simulink model "pllEncoder"  (R2024b)
settings: Solver=FixedStepAuto  StartTime=0.0  StopTime=Tend  FixedStep=0.0001  RelTol=1e-4
values from neighbouring files (symbols this model uses):
  pole_1_Hz = -10    [computing_speed.m]    (also in setup.m)
  pole_2_Hz = -100    [computing_speed.m]    (also in setup.m)
  Ts = 1e-4    (= 0.0001)    [setup.m]    (also in test.m = 0.001)
undefined symbols (not defined in the file or in its folder): DiscIntNeverNeededParam
settings Model: Creator=puroh  LastModifiedBy=tnoguchi
settings DataIOCC: SaveOutput=off  SaveTime=off
settings OptimizationCC: DefaultParameterBehavior=Inlined  EnhancedBackFolding=on  PassReuseOutputArgsAs=Individual arguments  ZeroExternalMemoryAtStartup=off  ZeroInternalMemoryAtStartup=off  OptimizeBlockOrder=speed  DifferentSizesBufferReuse=on  EfficientTunableParamExpr=on
settings DebuggingCC: ParameterTunabilityLossMsg=error  UnconnectedInputMsg=warning  UnconnectedOutputMsg=warning  UnconnectedLineMsg=warning
settings ModelReferenceCC: EnableRefExpFcnMdlSchedulingChecks=on
settings SFSimCC: MATLABDynamicMemAlloc=off
settings RTWCC: Description=Embedded Coder  SystemTargetFile=ert.tlc  TemplateMakefile=ert_default_tmf  GPUComputeCapability=3.5  DLArmComputeVersion=19.05
settings CodeAppCC: ForceParamTrailComments=on  IgnoreCustomStorageClasses=off  OperatorAnnotations=on  SimulinkDataObjDesc=on  SFDataObjDesc=on  InsertBlockDesc=on
settings ERTTargetCC: TargetLangStandard=C99 (ISO)  ERTCustomFileTemplate=example_file_process.tlc  DynamicArrayContainerType=coder::array
settings ConfigComp: CovBoundaryAbsTol=1.0e-5

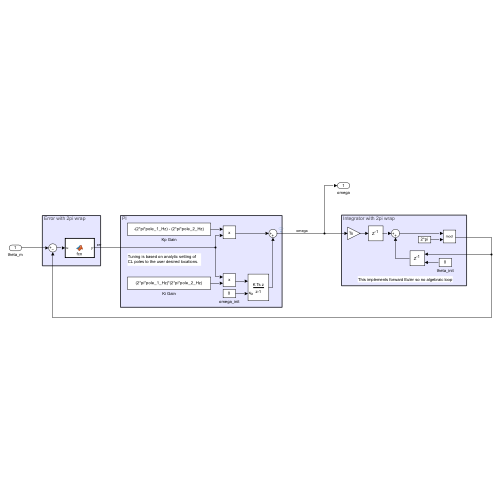
[thumbnail: Simulink's stored preview of the top-level diagram]
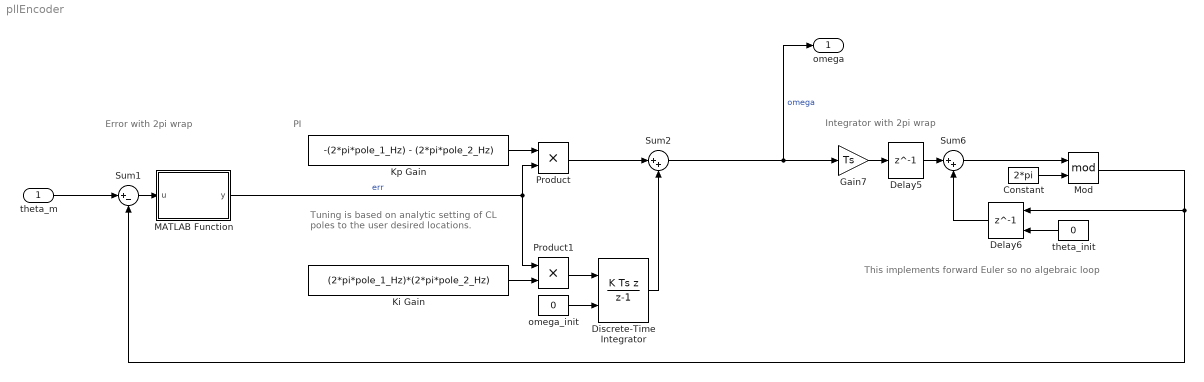
== system pllEncoder ==
  note: Tuning is based on analytic setting of CL poles to the user desired locations.
  note: PI
  note: Error with 2pi wrap
  note: Integrator with 2pi wrap
  note: This implements forward Euler so no algebraic loop
  theta_m : Inport  OutDataTypeStr=double  PortDimensions=1  SampleTime=[0.0001,0]
  Constant : Constant  Value=2*pi
  Delay5 : Delay  DelayLength=1  InputProcessing=Columns as channels (frame based)
  Delay6 : Delay  DelayLength=1  InitialConditionSource=Input port  InputProcessing=Columns as channels (frame based)
      settings: InputPortMap=u0,p4
  Discrete-Time Integrator : DiscreteIntegrator  IntegratorMethod=Integration: Backward Euler  InitialConditionSource=external  SampleTime=-1  ICPrevOutput=DiscIntNeverNeededParam  ICPrevScaledInput=DiscIntNeverNeededParam
  Gain7 : Gain  Gain=Ts
  Ki Gain : Constant  Value=(2*pi*pole_1_Hz)*(2*pi*pole_2_Hz)
  Kp Gain : Constant  Value=-(2*pi*pole_1_Hz) - (2*pi*pole_2_Hz)
  MATLAB Function : MATLAB Function  TreatAsAtomicUnit=on
  Mod : Math  Operator=mod
  Product : Product
  Product1 : Product
  Sum1 : Sum  Inputs=|+-
  Sum2 : Sum  Inputs=|++
  Sum6 : Sum  Inputs=|++
  omega_init : Constant  Value=0
  theta_init : Constant  Value=0
  omega : Outport  OutDataTypeStr=double  PortDimensions=1  SampleTime=[0.0001,0]
  wires:
  Discrete-Time Integrator/1 -> Sum2/2
  Ki Gain/1 -> Product1/2
  Kp Gain/1 -> Product/1
  Sum6/1 -> Mod/1
  Mod/1 -> Delay6/1, Sum1/2
  Sum1/1 -> MATLAB Function/1(u)
  Delay5/1 -> Sum6/1
  omega_init/1 -> Discrete-Time Integrator/2
  theta_m/1 -> Sum1/1
  Gain7/1 -> Delay5/1
  Delay6/1 -> Sum6/2
  Constant/1 -> Mod/2
  theta_init/1 -> Delay6/2
  Product1/1 -> Discrete-Time Integrator/1
  MATLAB Function/1(y) -> Product/2, Product1/1  "err"
  Product/1 -> Sum2/1
  Sum2/1 -> omega/1, Gain7/1  "omega"

== matlab function pllEncoder/MATLAB Function ==
  data: u input; y output
function y = fcn(u)

y = u;

if y > pi
    y = y - 2*pi;
end

if y < -pi
    y = y + 2*pi;
end
